simulink model "PoliArd_PID_track_2015a"  (R2015a)
settings: Solver=ode3  StartTime=0.0  StopTime=inf  FixedStep=0.001  RelTol=1e-3
values from neighbouring files (symbols this model uses):
  b = 0.0245    [Main_PoliArd_PID_track.m]
  cx = [1.83578189847e-05 0.000815203238403]    [calibration.mat]
  cy = [1.80605123685e-05 -0.00194285103796]    [calibration.mat]
  T_circle = 2    [Main_PoliArd_PID_track.m]
undefined symbols (not defined in the file or in its folder): KIy, KPy
libraries: PoliArd x10, simulink x3, simulink_extras x2
settings Model: CovHtmlReporting=off  ExtModeTrigDuration=2  Creator=User  LastModifiedBy=vise
settings OptimizationCC: LifeSpan=1
settings DebuggingCC: UnderspecifiedInitializationDetection=Classic  MergeDetectMultiDrivingBlocksExec=none
settings HardwareCC: ProdLargestAtomicInteger=Long  ProdLargestAtomicFloat=Double  ProdEndianess=LittleEndian  ProdHWDeviceType=ARM Compatible->ARM Cortex
settings RTWCC: SystemTargetFile=realtime.tlc  GenerateMakefile=off  TemplateMakefile=realtime.tmf  Description=Run on Target Hardware  RTWVerbose=off
settings ERTTargetCC: CombineOutputUpdateFcns=off  ExtModeTransport=3  ExtModeMexFile=ext_serial_win32_comm_rtt  ExtModeMexArgs=0 1 9600  InlinedParameterPlacement=Hierarchical  ERTSrcFileBannerTemplate=realtime_code_template.cgt  ERTHdrFileBannerTemplate=realtime_code_template.cgt  ERTDataSrcFileTemplate=realtime_code_template.cgt  ERTDataHdrFileTemplate=realtime_code_template.cgt  ERTCustomFileTemplate=realtime_file_process.tlc

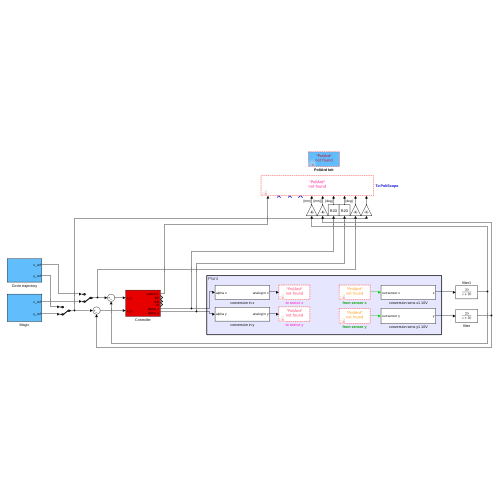
[thumbnail: Simulink's stored preview of the top-level diagram]
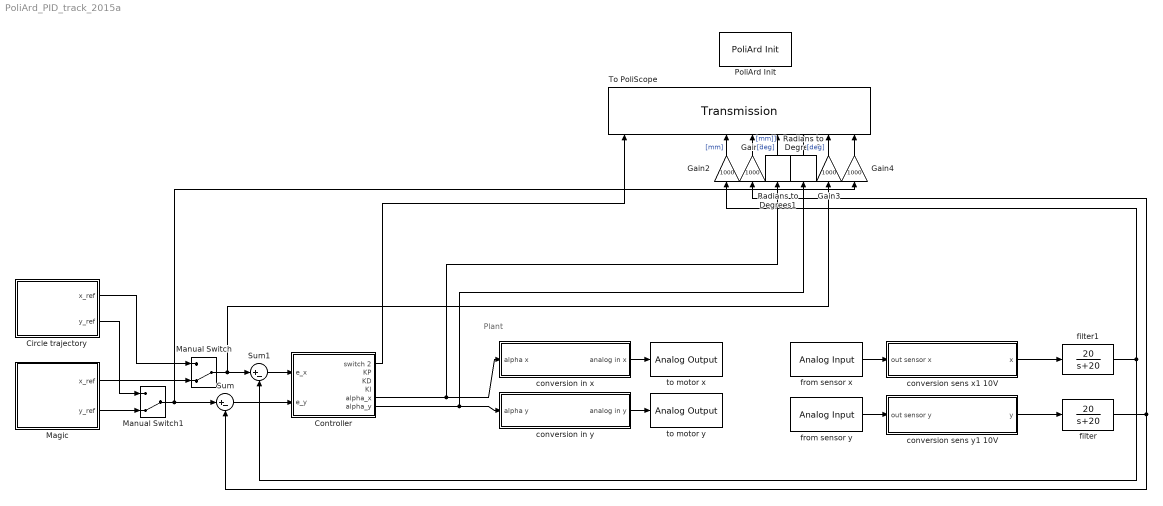
== system PoliArd_PID_track_2015a ==
  note: Plant
  Circle trajectory : Subsystem
  Controller : Subsystem
  Gain{1..4} (4 alike) : Gain  Gain=1000
  Magic : Subsystem
  Manual Switch : ManualSwitch  CurrentSetting=0
  Manual Switch1 : ManualSwitch  CurrentSetting=0
  PoliArd Init : PoliArd/PoliArd Init
  Radians to Degrees1 : simulink_extras/Transformations/Radians to Degrees
  Radians to Degrees2 : simulink_extras/Transformations/Radians to Degrees
  Sum : Sum  Inputs=|+-
  Sum1 : Sum  Inputs=|+-
  To PoliScope : PoliArd/Transmission  sample_freq=1000  sig_to_send=6
  conversion in x : Subsystem
  conversion in y : Subsystem
  conversion sens x1 10V : Subsystem
  conversion sens y1 10V : Subsystem
  filter : TransferFcn  Numerator=[20]  Denominator=[1 20]
  filter1 : TransferFcn  Numerator=[20]  Denominator=[1 20]
  from sensor x : PoliArd/Analog Input  AIpin_mask=4  AIsample=-1
  from sensor y : PoliArd/Analog Input  AIpin_mask=3  AIsample=-1
  to motor x : PoliArd/Analog Output  DAC_pin_mask=1
  to motor y : PoliArd/Analog Output  DAC_pin_mask=2
  wires:
  filter/1 -> Sum/2, Gain1/1
  filter1/1 -> Sum1/2, Gain2/1
  Gain1/1 -> To PoliScope/6  "[mm]]"
  Gain2/1 -> To PoliScope/5  "[mm]"
  from sensor x/1 -> conversion sens x1 10V/1(out sensor x)
  from sensor y/1 -> conversion sens y1 10V/1(out sensor y)
  conversion in x/1(analog in x) -> to motor x/1
  conversion in y/1(analog in y) -> to motor y/1
  conversion sens x1 10V/1(x) -> filter1/1
  conversion sens y1 10V/1(y) -> filter/1
  Sum/1 -> Controller/2(e_y)
  Sum1/1 -> Controller/1(e_x)
  Magic/1(x_ref) -> Manual Switch/2
  Magic/2(y_ref) -> Manual Switch1/2
  Controller/1("switch 2 ") -> To PoliScope/1
  Controller/5(alpha_x) -> Radians to Degrees1/1, conversion in x/1(alpha x)
  Controller/6(alpha_y) -> Radians to Degrees2/1, conversion in y/1(alpha y)
  Manual Switch/1 -> Gain3/1, Sum1/1
  Manual Switch1/1 -> Sum/1, Gain4/1
  Circle trajectory/1(x_ref) -> Manual Switch/1
  Circle trajectory/2(y_ref) -> Manual Switch1/1
  Radians to Degrees1/1 -> To PoliScope/7  "[deg]"
  Radians to Degrees2/1 -> To PoliScope/8  "[deg]"
  Gain3/1 -> To PoliScope/9
  Gain4/1 -> To PoliScope/10

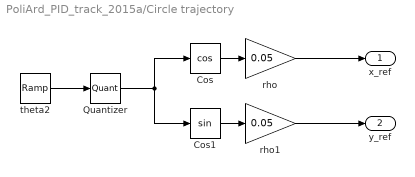
== system PoliArd_PID_track_2015a/Circle trajectory ==
  Cos : Trigonometry  Operator=cos
  Cos1 : Trigonometry
  Quantizer : Quantizer  QuantizationInterval=0.001
  rho : Gain  Gain=0.05
  rho1 : Gain  Gain=0.05
  theta2 : simulink/Sources/Ramp  slope=2*pi/T_circle  start=0  X0=0
  x_ref : Outport
  y_ref : Outport  Port=2
  wires:
  Cos/1 -> rho/1
  Cos1/1 -> rho1/1
  rho1/1 -> y_ref/1
  rho/1 -> x_ref/1
  theta2/1 -> Quantizer/1
  Quantizer/1 -> Cos1/1, Cos/1

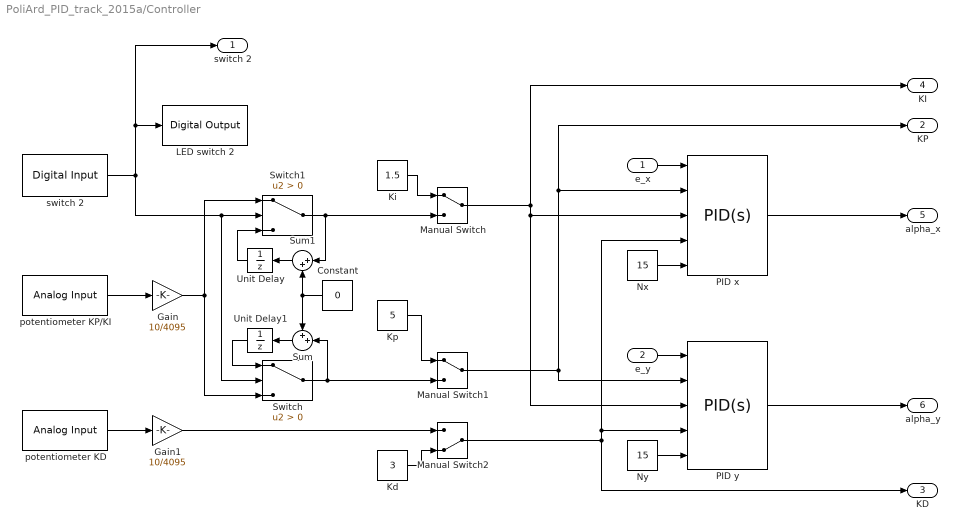
== system PoliArd_PID_track_2015a/Controller ==
  e_x : Inport
  e_y : Inport  Port=2
  Constant : Constant  Value=0
  Gain : Gain  Gain=10/4095
  Gain1 : Gain  Gain=10/4095
  "Kd " : Constant  Value=3
  Ki : Constant  Value=1.5
  Kp : Constant  Value=5
  "LED switch 2 " : PoliArd/Digital Output  DO_pin=1
  Manual Switch : ManualSwitch
  Manual Switch1 : ManualSwitch
  Manual Switch2 : ManualSwitch  CurrentSetting=0
  Nx : Constant  Value=15
  Ny : Constant  Value=15
  PID x : simulink/Continuous/PID Controller  Controller=PID  Form=Parallel  TimeDomain=Continuous-time  SampleTime=-1  IntegratorMethod=Forward Euler  FilterMethod=Forward Euler  ControllerParametersSource=external  P=5  I=2  D=6  N=30  UseFilter=on  InitialConditionSource=internal  InitialConditionForIntegrator=0  InitialConditionForFilter=0  DifferentiatorICPrevScaledInput=0  ExternalReset=none  TrackingMode=off  Kt=1  LimitOutput=on  UpperSaturationLimit=deg2rad(75)  LowerSaturationLimit=deg2rad(-75)  LinearizeAsGain=on  AntiWindupMode=back-calculation  Kb=0.8  POutMin=[]  POutMax=[]  IOutMin=[]  IOutMax=[]  DOutMin=[]  DOutMax=[]  NOutMin=[]  NOutMax=[]  SumOutMin=[]  SumOutMax=[]  SaturationOutMin=[]  SaturationOutMax=[]  PParamMin=[]  PParamMax=[]  IParamMin=[]  IParamMax=[]  DParamMin=[]  DParamMax=[]  NParamMin=[]  NParamMax=[]  KbParamMin=[]  KbParamMax=[]  KtParamMin=[]  KtParamMax=[]  KbOutMin=[]  KbOutMax=[]  KtOutMin=[]  KtOutMax=[]  IntegratorOutMin=[]  IntegratorOutMax=[]  FilterOutMin=[]  FilterOutMax=[]  SumI1OutMin=[]  SumI1OutMax=[]  SumI2OutMin=[]  SumI2OutMax=[]  SumI3OutMin=[]  SumI3OutMax=[]  SumDOutMin=[]  SumDOutMax=[]  DifferentiatorOutMin=[]  DifferentiatorOutMax=[]  IntegratorContinuousStateAttributes=''  IntegratorStateMustResolveToSignalObject=off  IntegratorRTWStateStorageClass=Auto  FilterContinuousStateAttributes=''  FilterStateMustResolveToSignalObject=off  FilterRTWStateStorageClass=Auto
  PID y : simulink/Continuous/PID Controller  Controller=PID  Form=Parallel  TimeDomain=Continuous-time  SampleTime=-1  IntegratorMethod=Forward Euler  FilterMethod=Forward Euler  ControllerParametersSource=external  P=KPy  I=KIy  D=-0.189219016325203  N=1.72044274974478  UseFilter=on  InitialConditionSource=internal  InitialConditionForIntegrator=0  InitialConditionForFilter=0  DifferentiatorICPrevScaledInput=0  ExternalReset=none  TrackingMode=off  Kt=1  LimitOutput=on  UpperSaturationLimit=deg2rad(45)  LowerSaturationLimit=deg2rad(-45)  LinearizeAsGain=on  AntiWindupMode=back-calculation  Kb=0.8  POutMin=[]  POutMax=[]  IOutMin=[]  IOutMax=[]  DOutMin=[]  DOutMax=[]  NOutMin=[]  NOutMax=[]  SumOutMin=[]  SumOutMax=[]  SaturationOutMin=[]  SaturationOutMax=[]  PParamMin=[]  PParamMax=[]  IParamMin=[]  IParamMax=[]  DParamMin=[]  DParamMax=[]  NParamMin=[]  NParamMax=[]  KbParamMin=[]  KbParamMax=[]  KtParamMin=[]  KtParamMax=[]  KbOutMin=[]  KbOutMax=[]  KtOutMin=[]  KtOutMax=[]  IntegratorOutMin=[]  IntegratorOutMax=[]  FilterOutMin=[]  FilterOutMax=[]  SumI1OutMin=[]  SumI1OutMax=[]  SumI2OutMin=[]  SumI2OutMax=[]  SumI3OutMin=[]  SumI3OutMax=[]  SumDOutMin=[]  SumDOutMax=[]  DifferentiatorOutMin=[]  DifferentiatorOutMax=[]  IntegratorContinuousStateAttributes=''  IntegratorStateMustResolveToSignalObject=off  IntegratorRTWStateStorageClass=Auto  FilterContinuousStateAttributes=''  FilterStateMustResolveToSignalObject=off  FilterRTWStateStorageClass=Auto
  Sum : Sum  Inputs=++|
  Sum1 : Sum  Inputs=|++
  Switch : Switch  Criteria=u2 > Threshold
  Switch1 : Switch  Criteria=u2 > Threshold
  Unit Delay : UnitDelay  SampleTime=-1  HasFrameUpgradeWarning=on
  Unit Delay1 : UnitDelay  SampleTime=-1  HasFrameUpgradeWarning=on
  potentiometer KD : PoliArd/Analog Input  AIpin_mask=9  AIsample=-1
  potentiometer KP/KI : PoliArd/Analog Input  AIpin_mask=8  AIsample=-1
  switch 2 : PoliArd/Digital Input  DI_pin=2  DIsample=-1
  "switch 2 " : Outport
  KP : Outport  Port=2
  KD : Outport  Port=3
  KI : Outport  Port=4
  alpha_x : Outport  Port=5
  alpha_y : Outport  Port=6
  wires:
  "Kd "/1 -> Manual Switch2/2
  Manual Switch2/1 -> PID x/4, PID y/4, KD/1
  Gain1/1 -> Manual Switch2/1
  Manual Switch1/1 -> PID y/2, KP/1, PID x/2
  Kp/1 -> Manual Switch1/1
  Ki/1 -> Manual Switch/1
  Manual Switch/1 -> PID y/3, PID x/3, KI/1
  Unit Delay1/1 -> Switch/1
  Unit Delay/1 -> Switch1/3
  Sum1/1 -> Unit Delay/1
  Constant/1 -> Sum/1, Sum1/2
  Sum/1 -> Unit Delay1/1
  switch 2/1 -> Switch1/2, Switch/2, "LED switch 2 "/1, "switch 2 "/1
  Switch/1 -> Manual Switch1/2, Sum/2
  Ny/1 -> PID y/5
  Nx/1 -> PID x/5
  e_y/1 -> PID y/1
  e_x/1 -> PID x/1
  Switch1/1 -> Sum1/1, Manual Switch/2
  Gain/1 -> Switch/3, Switch1/1
  potentiometer KP/KI/1 -> Gain/1
  potentiometer KD/1 -> Gain1/1
  PID x/1 -> alpha_x/1
  PID y/1 -> alpha_y/1

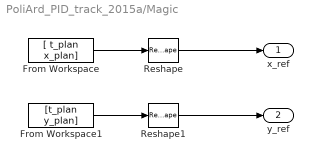
== system PoliArd_PID_track_2015a/Magic ==
  From Workspace : FromWorkspace  VariableName=[ t_plan x_plan]  OutputAfterFinalValue=Holding final value
  From Workspace1 : FromWorkspace  VariableName=[t_plan y_plan]  OutputAfterFinalValue=Holding final value
  Reshape : Reshape  OutputDimensionality=Column vector (2-D)
  Reshape1 : Reshape  OutputDimensionality=Column vector (2-D)
  x_ref : Outport
  y_ref : Outport  Port=2
  wires:
  Reshape/1 -> x_ref/1
  Reshape1/1 -> y_ref/1
  From Workspace/1 -> Reshape/1
  From Workspace1/1 -> Reshape1/1

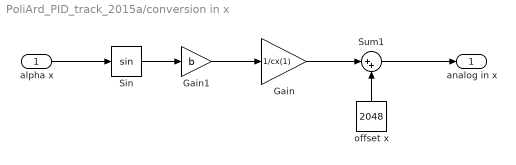
== system PoliArd_PID_track_2015a/conversion in x ==
  alpha x : Inport
  Gain : Gain  Gain=1/cx(1)
  Gain1 : Gain  Gain=b
  Sin : Trigonometry
  Sum1 : Sum  Inputs=|++
  offset x : Constant  Value=2048
  analog in x : Outport
  wires:
  Sin/1 -> Gain1/1
  Gain1/1 -> Gain/1
  Gain/1 -> Sum1/1
  Sum1/1 -> analog in x/1
  offset x/1 -> Sum1/2
  alpha x/1 -> Sin/1

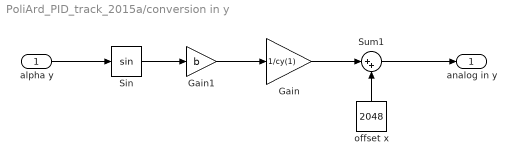
== system PoliArd_PID_track_2015a/conversion in y ==
  alpha y : Inport
  Gain : Gain  Gain=1/cy(1)
  Gain1 : Gain  Gain=b
  Sin : Trigonometry
  Sum1 : Sum  Inputs=|++
  offset x : Constant  Value=2048
  analog in y : Outport
  wires:
  alpha y/1 -> Sin/1
  offset x/1 -> Sum1/2
  Sum1/1 -> analog in y/1
  Gain/1 -> Sum1/1
  Gain1/1 -> Gain/1
  Sin/1 -> Gain1/1

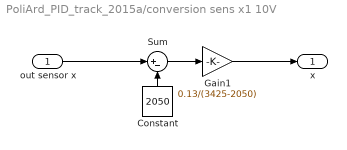
== system PoliArd_PID_track_2015a/conversion sens x1 10V ==
  out sensor x : Inport
  Constant : Constant  Value=2050
  Gain1 : Gain  Gain=0.13/(3425-2050)
  Sum : Sum  Inputs=|+-
  x : Outport
  wires:
  Gain1/1 -> x/1
  out sensor x/1 -> Sum/1
  Sum/1 -> Gain1/1
  Constant/1 -> Sum/2

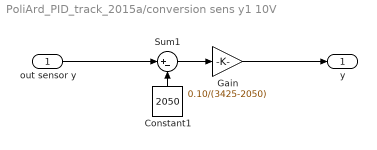
== system PoliArd_PID_track_2015a/conversion sens y1 10V ==
  out sensor y : Inport
  Constant1 : Constant  Value=2050
  Gain : Gain  Gain=0.10/(3425-2050)
  Sum1 : Sum  Inputs=|+-
  y : Outport
  wires:
  Gain/1 -> y/1
  Constant1/1 -> Sum1/2
  Sum1/1 -> Gain/1
  out sensor y/1 -> Sum1/1
